simulink library "LIB_TF_G_112"  (Simulink 8.6)
settings: Solver=ode45  StartTime=0.0  StopTime=10.0  RelTol=1e-3
PreLoadFcn:
  | if exist('tl_preloadfcn','file'), tl_preloadfcn(gcs,402); end
PostLoadFcn:
  | if exist('tl_postloadfcn','file'), tl_postloadfcn(gcs,402); end
undefined symbols (not defined in the file): ddv, u2, u3
libraries: tllib x3
(part 3 of 4)

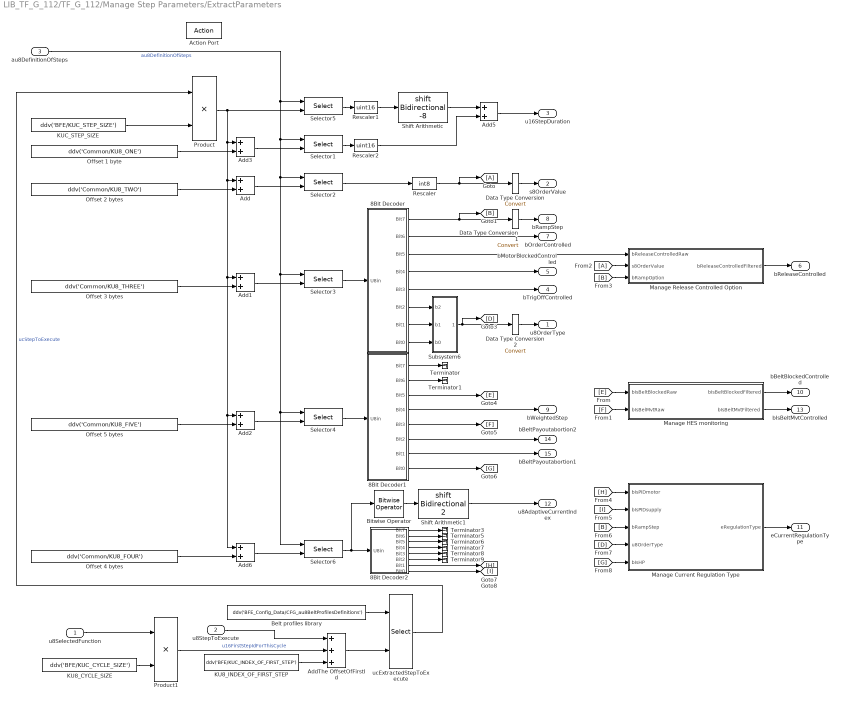
== system LIB_TF_G_112/TF_G_112/Manage Step Parameters/ExtractParameters ==
  u8SelectedFunction : Inport
  u8StepToExecute : Inport  Port=2
  au8DefinitionOfSteps : Inport  RequirementInfo={} %GIDa_5af58792_1cc9_4ce4_bae0_9036b424a801  Port=3
  Action Port : ActionPort  RequirementInfo={} %GIDa_b716945c_1562_44da_9f85_7ecf343fa6e8
  8Bit Decoder : Subsystem  RequirementInfo={} %GIDa_feba0c62_931c_4072_b0ff_45aba4007524  mask(TLSAMPLES_8BIT_DECODER){}
      mask help:
      | Decodes one UInt8 byte into 8 bits.
      | All inputs are boolean variables.
      |
      | Sample implementation using TargetLink Custom Code block.
      | Version 1.0.
  8Bit Decoder1 : Subsystem  RequirementInfo={} %GIDa_d8b7cbf2_0e68_4179_ae19_c2248359c39e  mask(TLSAMPLES_8BIT_DECODER){}
      mask help:
      | Decodes one UInt8 byte into 8 bits.
      | All inputs are boolean variables.
      |
      | Sample implementation using TargetLink Custom Code block.
      | Version 1.0.
  8Bit Decoder2 : Subsystem  RequirementInfo={} %GIDa_1ebe05c3_ad94_48a6_9eed_8520aa55f6d4  mask(TLSAMPLES_8BIT_DECODER){}
      mask help:
      | Decodes one UInt8 byte into 8 bits.
      | All inputs are boolean variables.
      |
      | Sample implementation using TargetLink Custom Code block.
      | Version 1.0.
  Add : Sum  RequirementInfo={} %GIDa_0a57a462_dd82_4f66_b861_c0720a7e3696  mask(TL_Sum){data={'output',{'name','u16StepByte2','type','UInt16'},'date',735951.66828546301}}
      settings: CopyFcn=if exist('tl_reset_reviewflag','file')==2,tl_reset_reviewflag(gcbh);end  DeleteFcn=if exist('delete_tlblock','file')==2,delete_tlblock(gcbh);end  NameChangeFcn=if exist('rename_tlblock','file')==2,rename_tlblock(gcbh);end  OpenFcn=if exist('tl_open_blockdlg','file')==2,tl_open_blockdlg(gcbh);else,open_system(gcbh,'parameter');end
      mask Help: eval(['if exist(''tl_online_help'',''file'') == 2, tl_online_help(''Topic'',''TL_Sum''),else, web([''jar:file:///'',matlabroot,''/help/toolbox/simulink/help.jar!/slref/' lower(get_param(gcbh,'Blocktype')) '.html''], ''-helpbrowser''),end'])
      mask Display: plot([-0.05, 1.05, NaN, -0.05, 1.05],[.01, .01, NaN, .99, .99])
  Add1 : Sum  RequirementInfo={} %GIDa_51ab638f_d75f_42d5_a1b3_c6f4ae26db52  mask(TL_Sum){data={'output',{'name','u16StepByte3','type','UInt16'},'date',735951.66828510421}}
      settings: CopyFcn=if exist('tl_reset_reviewflag','file')==2,tl_reset_reviewflag(gcbh);end  DeleteFcn=if exist('delete_tlblock','file')==2,delete_tlblock(gcbh);end  NameChangeFcn=if exist('rename_tlblock','file')==2,rename_tlblock(gcbh);end  OpenFcn=if exist('tl_open_blockdlg','file')==2,tl_open_blockdlg(gcbh);else,open_system(gcbh,'parameter');end
      mask Help: eval(['if exist(''tl_online_help'',''file'') == 2, tl_online_help(''Topic'',''TL_Sum''),else, web([''jar:file:///'',matlabroot,''/help/toolbox/simulink/help.jar!/slref/' lower(get_param(gcbh,'Blocktype')) '.html''], ''-helpbrowser''),end'])
      mask Display: plot([-0.05, 1.05, NaN, -0.05, 1.05],[.01, .01, NaN, .99, .99])
  Add2 : Sum  RequirementInfo={} %GIDa_81f2c18e_91ec_4878_8faa_bc376be4849a  mask(TL_Sum){data={'output',{'name','u16StepByte5','type','UInt16'},'date',735951.66828473378}}
      settings: CopyFcn=if exist('tl_reset_reviewflag','file')==2,tl_reset_reviewflag(gcbh);end  DeleteFcn=if exist('delete_tlblock','file')==2,delete_tlblock(gcbh);end  NameChangeFcn=if exist('rename_tlblock','file')==2,rename_tlblock(gcbh);end  OpenFcn=if exist('tl_open_blockdlg','file')==2,tl_open_blockdlg(gcbh);else,open_system(gcbh,'parameter');end
      mask Help: eval(['if exist(''tl_online_help'',''file'') == 2, tl_online_help(''Topic'',''TL_Sum''),else, web([''jar:file:///'',matlabroot,''/help/toolbox/simulink/help.jar!/slref/' lower(get_param(gcbh,'Blocktype')) '.html''], ''-helpbrowser''),end'])
      mask Display: plot([-0.05, 1.05, NaN, -0.05, 1.05],[.01, .01, NaN, .99, .99])
  Add3 : Sum  RequirementInfo={} %GIDa_b8557759_ab8c_4963_8e82_441dee7d1691  mask(TL_Sum){data={'output',{'name','u16StepByte1','type','UInt16'},'date',735951.66828436346}}
      settings: CopyFcn=if exist('tl_reset_reviewflag','file')==2,tl_reset_reviewflag(gcbh);end  DeleteFcn=if exist('delete_tlblock','file')==2,delete_tlblock(gcbh);end  NameChangeFcn=if exist('rename_tlblock','file')==2,rename_tlblock(gcbh);end  OpenFcn=if exist('tl_open_blockdlg','file')==2,tl_open_blockdlg(gcbh);else,open_system(gcbh,'parameter');end
      mask Help: eval(['if exist(''tl_online_help'',''file'') == 2, tl_online_help(''Topic'',''TL_Sum''),else, web([''jar:file:///'',matlabroot,''/help/toolbox/simulink/help.jar!/slref/' lower(get_param(gcbh,'Blocktype')) '.html''], ''-helpbrowser''),end'])
      mask Display: plot([-0.05, 1.05, NaN, -0.05, 1.05],[.01, .01, NaN, .99, .99])
  Add5 : Sum  Description=Requirement Titi  RequirementInfo={'other' '..\..\..\..\Documents and Settings\cedric.sauvage\Desktop\BFE_Design.doc' '@Simulink_requirement_item_2' 'true' 'DSG_BFE_00026' '' } %GIDa_05628d3b_8b03_4e96_b55e_ea34f4ea1d4e  AccumDataTypeStr=uint16  OutDataTypeStr=uint16  mask(TL_Sum){data={'comment',{'text',['[COVERS: DSG_BFE_00026]'],'placement',2},'output',{'type','UInt16'},'date',735951.6682839815}}
      settings: CopyFcn=if exist('tl_reset_reviewflag','file')==2,tl_reset_reviewflag(gcbh);end  DeleteFcn=if exist('delete_tlblock','file')==2,delete_tlblock(gcbh);end  NameChangeFcn=if exist('rename_tlblock','file')==2,rename_tlblock(gcbh);end  OpenFcn=if exist('tl_open_blockdlg','file')==2,tl_open_blockdlg(gcbh);else,open_system(gcbh,'parameter');end
      mask Help: eval(['if exist(''tl_online_help'',''file'') == 2, tl_online_help(''Topic'',''TL_Sum''),else, web([''jar:file:///'',matlabroot,''/help/toolbox/simulink/help.jar!/slref/' lower(get_param(gcbh,'Blocktype')) '.html''], ''-helpbrowser''),end'])
      mask Display: plot([-0.05, 1.05, NaN, -0.05, 1.05],[.01, .01, NaN, .99, .99])
  Add6 : Sum  RequirementInfo={} %GIDa_a90a7fc2_4cf2_40a8_9795_cd5c47b64498  mask(TL_Sum){data={'output',{'name','u16StepByte4','type','UInt16'},'date',735951.66828361107}}
      settings: CopyFcn=if exist('tl_reset_reviewflag','file')==2,tl_reset_reviewflag(gcbh);end  DeleteFcn=if exist('delete_tlblock','file')==2,delete_tlblock(gcbh);end  NameChangeFcn=if exist('rename_tlblock','file')==2,rename_tlblock(gcbh);end  OpenFcn=if exist('tl_open_blockdlg','file')==2,tl_open_blockdlg(gcbh);else,open_system(gcbh,'parameter');end
      mask Help: eval(['if exist(''tl_online_help'',''file'') == 2, tl_online_help(''Topic'',''TL_Sum''),else, web([''jar:file:///'',matlabroot,''/help/toolbox/simulink/help.jar!/slref/' lower(get_param(gcbh,'Blocktype')) '.html''], ''-helpbrowser''),end'])
      mask Display: plot([-0.05, 1.05, NaN, -0.05, 1.05],[.01, .01, NaN, .99, .99])
  AddThe OffsetOfFirstId : Sum  RequirementInfo={} %GIDa_cb935c7f_f3b5_47b3_8f86_966f4978fe65  Inputs=+++  SaturateOnIntegerOverflow=on  OutDataTypeStr=Inherit: Same as first input  mask(TL_Sum){data={'output',{'name','u16StepBytePosition','class','MERGEABLE_GLOBAL_ASR4','type','UInt16'},'date',736468.40163105319}}
      settings: CopyFcn=if exist('tl_reset_reviewflag','file')==2,tl_reset_reviewflag(gcbh);end  DeleteFcn=if exist('delete_tlblock','file')==2,delete_tlblock(gcbh);end  NameChangeFcn=if exist('rename_tlblock','file')==2,rename_tlblock(gcbh);end  OpenFcn=if exist('tl_open_blockdlg','file')==2,tl_open_blockdlg(gcbh);else,open_system(gcbh,'parameter');end
      mask Help: eval(['if exist(''tl_online_help'',''file'') == 2, tl_online_help(''Topic'',''TL_Sum''),else, web([''jar:file:///'',matlabroot,''/help/toolbox/simulink/help.jar!/slref/' lower(get_param(gcbh,'Blocktype')) '.html''], ''-helpbrowser''),end'])
      mask Display: plot([-0.05, 1.05, NaN, -0.05, 1.05],[.01, .01, NaN, .99, .99])
  Belt profiles library : Constant  RequirementInfo={} %GIDa_12d42078_1b0f_4eb4_abcd_54e33e78707a  Value=ddv('BFE_Config_Data/CFG_au8BeltProfilesDefinitions')  OutDataTypeStr=uint8  SampleTime=-1  mask(TL_Constant){data={'output',{'variable','BFE_Config_Data/CFG_au8BeltProfilesDefinitions'},'autoscaling',{'mode',2,'scalingvalid',1},'date',735951.66828289349}}
      settings: CopyFcn=if exist('tl_reset_reviewflag','file')==2,tl_reset_reviewflag(gcbh);end  DeleteFcn=if exist('delete_tlblock','file')==2,delete_tlblock(gcbh);end  NameChangeFcn=if exist('rename_tlblock','file')==2,rename_tlblock(gcbh);end  OpenFcn=if exist('tl_open_blockdlg','file')==2,tl_open_blockdlg(gcbh);else,open_system(gcbh,'parameter');end
      mask Help: eval(['if exist(''tl_online_help'',''file'') == 2, tl_online_help(''Topic'',''TL_Constant''),else, web([''jar:file:///'',matlabroot,''/help/toolbox/simulink/help.jar!/slref/' lower(get_param(gcbh,'Blocktype')) '.html''], ''-helpbrowser''),end'])
      mask Display: plot([-0.05, 1.05, NaN, -0.05, 1.05],[.01, .01, NaN, .99, .99])
  Bitwise Operator : tllib/Bitwise Operator  logicop=AND  UseBitMask=on  BitMask=bin2dec('11111100')  BitMaskRealWorld=Stored Integer  data={'bitmask',{'variable','Common/KU8_MASK_BITS_2_7'},'date',735951.66828241898}
  Data Type Conversion : DataTypeConversion
  Data Type Conversion1 : DataTypeConversion
  Data Type Conversion2 : DataTypeConversion
  KU8_CYCLE_SIZE : Constant  RequirementInfo={} %GIDa_f33bf5cd_925c_4e93_b1c0_651200f97367  Value=ddv('BFE/KUC_CYCLE_SIZE')  OutDataTypeStr=Inherit: Inherit via back propagation  mask(TL_Constant){data={'output',{'variable','BFE/KUC_CYCLE_SIZE'},'date',735951.66828206019}}
      settings: CopyFcn=if exist('tl_reset_reviewflag','file')==2,tl_reset_reviewflag(gcbh);end  DeleteFcn=if exist('delete_tlblock','file')==2,delete_tlblock(gcbh);end  NameChangeFcn=if exist('rename_tlblock','file')==2,rename_tlblock(gcbh);end  OpenFcn=if exist('tl_open_blockdlg','file')==2,tl_open_blockdlg(gcbh);else,open_system(gcbh,'parameter');end
      mask Help: eval(['if exist(''tl_online_help'',''file'') == 2, tl_online_help(''Topic'',''TL_Constant''),else, web([''jar:file:///'',matlabroot,''/help/toolbox/simulink/help.jar!/slref/' lower(get_param(gcbh,'Blocktype')) '.html''], ''-helpbrowser''),end'])
      mask Display: plot([-0.05, 1.05, NaN, -0.05, 1.05],[.01, .01, NaN, .99, .99])
  KU8_INDEX_OF_FIRST_STEP : Constant  RequirementInfo={} %GIDa_c9f92c82_efc8_46a4_b98e_26be3633ccb9  Value=ddv('BFE/KUC_INDEX_OF_FIRST_STEP')  OutDataTypeStr=Inherit: Inherit via back propagation  mask(TL_Constant){data={'output',{'variable','BFE/KUC_INDEX_OF_FIRST_STEP'},'date',735951.66828170139}}
      settings: CopyFcn=if exist('tl_reset_reviewflag','file')==2,tl_reset_reviewflag(gcbh);end  DeleteFcn=if exist('delete_tlblock','file')==2,delete_tlblock(gcbh);end  NameChangeFcn=if exist('rename_tlblock','file')==2,rename_tlblock(gcbh);end  OpenFcn=if exist('tl_open_blockdlg','file')==2,tl_open_blockdlg(gcbh);else,open_system(gcbh,'parameter');end
      mask Help: eval(['if exist(''tl_online_help'',''file'') == 2, tl_online_help(''Topic'',''TL_Constant''),else, web([''jar:file:///'',matlabroot,''/help/toolbox/simulink/help.jar!/slref/' lower(get_param(gcbh,'Blocktype')) '.html''], ''-helpbrowser''),end'])
      mask Display: plot([-0.05, 1.05, NaN, -0.05, 1.05],[.01, .01, NaN, .99, .99])
  KUC_STEP_SIZE : Constant  RequirementInfo={} %GIDa_b75dc5a3_ad3f_404e_b74d_edddff931102  Value=ddv('BFE/KUC_STEP_SIZE')  OutDataTypeStr=Inherit: Inherit via back propagation  SampleTime=-1  mask(TL_Constant){data={'output',{'variable','BFE/KUC_STEP_SIZE'},'date',735951.6682813426}}
      settings: CopyFcn=if exist('tl_reset_reviewflag','file')==2,tl_reset_reviewflag(gcbh);end  DeleteFcn=if exist('delete_tlblock','file')==2,delete_tlblock(gcbh);end  NameChangeFcn=if exist('rename_tlblock','file')==2,rename_tlblock(gcbh);end  OpenFcn=if exist('tl_open_blockdlg','file')==2,tl_open_blockdlg(gcbh);else,open_system(gcbh,'parameter');end
      mask Help: eval(['if exist(''tl_online_help'',''file'') == 2, tl_online_help(''Topic'',''TL_Constant''),else, web([''jar:file:///'',matlabroot,''/help/toolbox/simulink/help.jar!/slref/' lower(get_param(gcbh,'Blocktype')) '.html''], ''-helpbrowser''),end'])
      mask Display: plot([-0.05, 1.05, NaN, -0.05, 1.05],[.01, .01, NaN, .99, .99])
  Manage Current Regulation Type : Subsystem  TreatAsAtomicUnit=on
  Manage HES monitoring : Subsystem  TreatAsAtomicUnit=on
  Manage Release Controlled Option : Subsystem  TreatAsAtomicUnit=on
  Offset 1 byte : Constant  RequirementInfo={} %GIDa_3a3d9ef6_6e74_4523_8795_3102c60b89ad  Value=ddv('Common/KU8_ONE')  OutDataTypeStr=uint8  SampleTime=-1  mask(TL_Constant){data={'output',{'variable','Common/KU8_ONE'},'date',735951.66827084485}}
      settings: CopyFcn=if exist('tl_reset_reviewflag','file')==2,tl_reset_reviewflag(gcbh);end  DeleteFcn=if exist('delete_tlblock','file')==2,delete_tlblock(gcbh);end  NameChangeFcn=if exist('rename_tlblock','file')==2,rename_tlblock(gcbh);end  OpenFcn=if exist('tl_open_blockdlg','file')==2,tl_open_blockdlg(gcbh);else,open_system(gcbh,'parameter');end
      mask Help: eval(['if exist(''tl_online_help'',''file'') == 2, tl_online_help(''Topic'',''TL_Constant''),else, web([''jar:file:///'',matlabroot,''/help/toolbox/simulink/help.jar!/slref/' lower(get_param(gcbh,'Blocktype')) '.html''], ''-helpbrowser''),end'])
      mask Display: plot([-0.05, 1.05, NaN, -0.05, 1.05],[.01, .01, NaN, .99, .99])
  Offset 2 bytes : Constant  RequirementInfo={} %GIDa_19184c90_6870_45c3_8db8_a8942b4be325  Value=ddv('Common/KU8_TWO')  OutDataTypeStr=uint8  SampleTime=-1  mask(TL_Constant){data={'output',{'variable','Common/KU8_TWO'},'date',735951.66827048606}}
      settings: CopyFcn=if exist('tl_reset_reviewflag','file')==2,tl_reset_reviewflag(gcbh);end  DeleteFcn=if exist('delete_tlblock','file')==2,delete_tlblock(gcbh);end  NameChangeFcn=if exist('rename_tlblock','file')==2,rename_tlblock(gcbh);end  OpenFcn=if exist('tl_open_blockdlg','file')==2,tl_open_blockdlg(gcbh);else,open_system(gcbh,'parameter');end
      mask Help: eval(['if exist(''tl_online_help'',''file'') == 2, tl_online_help(''Topic'',''TL_Constant''),else, web([''jar:file:///'',matlabroot,''/help/toolbox/simulink/help.jar!/slref/' lower(get_param(gcbh,'Blocktype')) '.html''], ''-helpbrowser''),end'])
      mask Display: plot([-0.05, 1.05, NaN, -0.05, 1.05],[.01, .01, NaN, .99, .99])
  Offset 3 bytes : Constant  RequirementInfo={} %GIDa_4ca9dd1f_f166_4945_8d3c_5d2b0f97e3a1  Value=ddv('Common/KU8_THREE')  OutDataTypeStr=uint8  SampleTime=-1  mask(TL_Constant){data={'output',{'variable','Common/KU8_THREE'},'date',735951.66827010422}}
      settings: CopyFcn=if exist('tl_reset_reviewflag','file')==2,tl_reset_reviewflag(gcbh);end  DeleteFcn=if exist('delete_tlblock','file')==2,delete_tlblock(gcbh);end  NameChangeFcn=if exist('rename_tlblock','file')==2,rename_tlblock(gcbh);end  OpenFcn=if exist('tl_open_blockdlg','file')==2,tl_open_blockdlg(gcbh);else,open_system(gcbh,'parameter');end
      mask Help: eval(['if exist(''tl_online_help'',''file'') == 2, tl_online_help(''Topic'',''TL_Constant''),else, web([''jar:file:///'',matlabroot,''/help/toolbox/simulink/help.jar!/slref/' lower(get_param(gcbh,'Blocktype')) '.html''], ''-helpbrowser''),end'])
      mask Display: plot([-0.05, 1.05, NaN, -0.05, 1.05],[.01, .01, NaN, .99, .99])
  Offset 4 bytes : Constant  RequirementInfo={} %GIDa_ea66cbc1_e91d_4821_b668_d6b79850c644  Value=ddv('Common/KU8_FOUR')  OutDataTypeStr=uint8  SampleTime=-1  mask(TL_Constant){data={'output',{'variable','Common/KU8_FOUR'},'date',735951.66826973378}}
      settings: CopyFcn=if exist('tl_reset_reviewflag','file')==2,tl_reset_reviewflag(gcbh);end  DeleteFcn=if exist('delete_tlblock','file')==2,delete_tlblock(gcbh);end  NameChangeFcn=if exist('rename_tlblock','file')==2,rename_tlblock(gcbh);end  OpenFcn=if exist('tl_open_blockdlg','file')==2,tl_open_blockdlg(gcbh);else,open_system(gcbh,'parameter');end
      mask Help: eval(['if exist(''tl_online_help'',''file'') == 2, tl_online_help(''Topic'',''TL_Constant''),else, web([''jar:file:///'',matlabroot,''/help/toolbox/simulink/help.jar!/slref/' lower(get_param(gcbh,'Blocktype')) '.html''], ''-helpbrowser''),end'])
      mask Display: plot([-0.05, 1.05, NaN, -0.05, 1.05],[.01, .01, NaN, .99, .99])
  Offset 5 bytes : Constant  RequirementInfo={} %GIDa_d7e3fc43_2c8c_428d_9f27_caf2b47de596  Value=ddv('Common/KU8_FIVE')  OutDataTypeStr=uint8  SampleTime=-1  mask(TL_Constant){data={'output',{'variable','Common/KU8_FIVE'},'date',735951.66826935182}}
      settings: CopyFcn=if exist('tl_reset_reviewflag','file')==2,tl_reset_reviewflag(gcbh);end  DeleteFcn=if exist('delete_tlblock','file')==2,delete_tlblock(gcbh);end  NameChangeFcn=if exist('rename_tlblock','file')==2,rename_tlblock(gcbh);end  OpenFcn=if exist('tl_open_blockdlg','file')==2,tl_open_blockdlg(gcbh);else,open_system(gcbh,'parameter');end
      mask Help: eval(['if exist(''tl_online_help'',''file'') == 2, tl_online_help(''Topic'',''TL_Constant''),else, web([''jar:file:///'',matlabroot,''/help/toolbox/simulink/help.jar!/slref/' lower(get_param(gcbh,'Blocktype')) '.html''], ''-helpbrowser''),end'])
      mask Display: plot([-0.05, 1.05, NaN, -0.05, 1.05],[.01, .01, NaN, .99, .99])
  Product : Product  RequirementInfo={} %GIDa_7eb561e5_5106_47b1_bccb_d25d321f907e  OutDataTypeStr=uint16  RndMeth=Zero  mask(TL_Product){data={'output',{'name','u16StepByte0','class','MERGEABLE_GLOBAL_ASR4','type','UInt16'},'date',736468.39839604171}}
      settings: CopyFcn=if exist('tl_reset_reviewflag','file')==2,tl_reset_reviewflag(gcbh);end  DeleteFcn=if exist('delete_tlblock','file')==2,delete_tlblock(gcbh);end  NameChangeFcn=if exist('rename_tlblock','file')==2,rename_tlblock(gcbh);end  OpenFcn=if exist('tl_open_blockdlg','file')==2,tl_open_blockdlg(gcbh);else,open_system(gcbh,'parameter');end
      mask Help: eval(['if exist(''tl_online_help'',''file'') == 2, tl_online_help(''Topic'',''TL_Product''),else, web([''jar:file:///'',matlabroot,''/help/toolbox/simulink/help.jar!/slref/' lower(get_param(gcbh,'Blocktype')) '.html''], ''-helpbrowser''),end'])
      mask Display: plot([-0.05, 1.05, NaN, -0.05, 1.05],[.01, .01, NaN, .99, .99])
  Product1 : Product  RequirementInfo={} %GIDa_7bc72bc7_7488_430d_ac37_90a0b87b4fce  SaturateOnIntegerOverflow=on  RndMeth=Zero  mask(TL_Product){data={'output',{'type','UInt16'},'date',735951.66826856486}}
      settings: CopyFcn=if exist('tl_reset_reviewflag','file')==2,tl_reset_reviewflag(gcbh);end  DeleteFcn=if exist('delete_tlblock','file')==2,delete_tlblock(gcbh);end  NameChangeFcn=if exist('rename_tlblock','file')==2,rename_tlblock(gcbh);end  OpenFcn=if exist('tl_open_blockdlg','file')==2,tl_open_blockdlg(gcbh);else,open_system(gcbh,'parameter');end
      mask Help: eval(['if exist(''tl_online_help'',''file'') == 2, tl_online_help(''Topic'',''TL_Product''),else, web([''jar:file:///'',matlabroot,''/help/toolbox/simulink/help.jar!/slref/' lower(get_param(gcbh,'Blocktype')) '.html''], ''-helpbrowser''),end'])
      mask Display: plot([-0.05, 1.05, NaN, -0.05, 1.05],[.01, .01, NaN, .99, .99])
  Rescaler : DataTypeConversion  RequirementInfo={'other' '..\..\..\..\Documents and Settings\cedric.sauvage\Desktop\BFE_Design.doc' '@Simulink_requirement_item_3' 'true' 'DSG_BFE_00025' '' } %GIDa_58362dca_0e5a_418f_af47_1f6b1fc37d26  OutDataTypeStr=int8  RndMeth=Zero  mask(TL_Rescaler){data={'comment',{'text',['[COVERS: DSG_BFE_00025]'],'placement',2},'output',{'name','s8StepOrderValue','type','Int8'},'date',735951.66826821759}}
      settings: DeleteFcn=if exist('delete_tlblock','file')==2,delete_tlblock(gcbh);end  NameChangeFcn=if exist('rename_tlblock','file')==2,rename_tlblock(gcbh);end  OpenFcn=if exist('tl_open_blockdlg','file')==2,tl_open_blockdlg(gcbh);else,open_system(gcbh,'parameter');end
      mask Help: eval(['if exist(''tl_online_help'',''file'') == 2, tl_online_help(''Topic'',''TL_Rescaler''),else, web([''jar:file:///'',matlabroot,''/help/toolbox/simulink/help.jar!/slref/' lower(get_param(gcbh,'Blocktype')) '.html''], ''-helpbrowser''),end'])
      mask Display: plot([-0.05, 1.05, NaN, -0.05, 1.05],[.01, .01, NaN, .99, .99])
  Rescaler1 : DataTypeConversion  OutDataTypeStr=uint16  SaturateOnIntegerOverflow=on  RndMeth=Zero  mask(TL_Rescaler){data={'output',{'type','UInt16'},'date',735951.66826790513}}
      settings: DeleteFcn=if exist('delete_tlblock','file')==2,delete_tlblock(gcbh);end  NameChangeFcn=if exist('rename_tlblock','file')==2,rename_tlblock(gcbh);end  OpenFcn=if exist('tl_open_blockdlg','file')==2,tl_open_blockdlg(gcbh);else,open_system(gcbh,'parameter');end
      mask Help: eval(['if exist(''tl_online_help'',''file'') == 2, tl_online_help(''Topic'',''TL_Rescaler''),else, web([''jar:file:///'',matlabroot,''/help/toolbox/simulink/help.jar!/slref/' lower(get_param(gcbh,'Blocktype')) '.html''], ''-helpbrowser''),end'])
      mask Display: plot([-0.05, 1.05, NaN, -0.05, 1.05],[.01, .01, NaN, .99, .99])
  Rescaler2 : DataTypeConversion  OutDataTypeStr=uint16  SaturateOnIntegerOverflow=on  RndMeth=Zero  mask(TL_Rescaler){data={'output',{'type','UInt16'},'date',735951.66826758103}}
      settings: DeleteFcn=if exist('delete_tlblock','file')==2,delete_tlblock(gcbh);end  NameChangeFcn=if exist('rename_tlblock','file')==2,rename_tlblock(gcbh);end  OpenFcn=if exist('tl_open_blockdlg','file')==2,tl_open_blockdlg(gcbh);else,open_system(gcbh,'parameter');end
      mask Help: eval(['if exist(''tl_online_help'',''file'') == 2, tl_online_help(''Topic'',''TL_Rescaler''),else, web([''jar:file:///'',matlabroot,''/help/toolbox/simulink/help.jar!/slref/' lower(get_param(gcbh,'Blocktype')) '.html''], ''-helpbrowser''),end'])
      mask Display: plot([-0.05, 1.05, NaN, -0.05, 1.05],[.01, .01, NaN, .99, .99])
  Selector1 : Selector  RequirementInfo={} %GIDa_4422b87b_5746_46e1_a326_9d16cdd82f03  IndexMode=Zero-based  IndexOptions=Index vector (port)  Indices=[1:10]  OutputSizes=1
  Selector2 : Selector  RequirementInfo={} %GIDa_4d9cfe24_d7c1_4186_b1de_afe3f89ce847  IndexMode=Zero-based  IndexOptions=Index vector (port)  Indices=[1:10]  OutputSizes=1
  Selector3 : Selector  RequirementInfo={} %GIDa_709804a5_dd5b_4c61_8f3f_1a0b2ad04ecf  IndexMode=Zero-based  IndexOptions=Index vector (port)  Indices=[1:10]  OutputSizes=1
  Selector4 : Selector  RequirementInfo={} %GIDa_f598d6e8_f893_4a7f_8905_585de03faa36  IndexMode=Zero-based  IndexOptions=Index vector (port)  Indices=[1:10]  OutputSizes=1
  Selector5 : Selector  RequirementInfo={} %GIDa_dd185a0d_3844_4a34_af71_6fb5e1e75326  IndexMode=Zero-based  IndexOptions=Index vector (port)  Indices=[1:10]  OutputSizes=1
  Selector6 : Selector  RequirementInfo={} %GIDa_61c5be39_750f_4521_8022_d14d6bd83ead  IndexMode=Zero-based  IndexOptions=Index vector (port)  Indices=[1:10]  OutputSizes=1
  Shift Arithmetic : ArithShift  LoadFcn=hBlOcK = gcbh; if strcmp(get_param(hBlOcK, 'LinkStatus'), 'resolved'), set_param(hBlOcK, 'LinkStatus', 'none'); set_param(hBlOcK, 'LoadFcn', ''); end; clear('hBlOcK');  BitShiftNumber=-8  mask(TL_ArithShift){data={'date',735951.66826726857}}
      settings: DeleteFcn=if exist('delete_tlblock','file')==2,delete_tlblock(gcbh);end  NameChangeFcn=if exist('rename_tlblock','file')==2,rename_tlblock(gcbh);end  OpenFcn=if exist('tl_open_blockdlg','file')==2,tl_open_blockdlg(gcbh);else,open_system(gcbh,'parameter');end
      mask Help: eval(['if exist(''tl_online_help'',''file'') == 2, tl_online_help(''Topic'',''TL_ArithShift''),else, web([''jar:file:///'',matlabroot,''/help/toolbox/simulink/help.jar!/slref/' lower(get_param(gcbh,'Blocktype')) '.html''], ''-helpbrowser''),end'])
      mask Display: plot([-0.05, 1.05, NaN, -0.05, 1.05],[.01, .01, NaN, .99, .99])
  Shift Arithmetic1 : ArithShift  LoadFcn=hBlOcK = gcbh; if strcmp(get_param(hBlOcK, 'LinkStatus'), 'resolved'), set_param(hBlOcK, 'LinkStatus', 'none'); set_param(hBlOcK, 'LoadFcn', ''); end; clear('hBlOcK');  BitShiftNumber=2  mask(TL_ArithShift){data={'date',735951.66826699069}}
      settings: DeleteFcn=if exist('delete_tlblock','file')==2,delete_tlblock(gcbh);end  NameChangeFcn=if exist('rename_tlblock','file')==2,rename_tlblock(gcbh);end  OpenFcn=if exist('tl_open_blockdlg','file')==2,tl_open_blockdlg(gcbh);else,open_system(gcbh,'parameter');end
      mask Help: eval(['if exist(''tl_online_help'',''file'') == 2, tl_online_help(''Topic'',''TL_ArithShift''),else, web([''jar:file:///'',matlabroot,''/help/toolbox/simulink/help.jar!/slref/' lower(get_param(gcbh,'Blocktype')) '.html''], ''-helpbrowser''),end'])
      mask Display: plot([-0.05, 1.05, NaN, -0.05, 1.05],[.01, .01, NaN, .99, .99])
  Subsystem6 : Subsystem  RequirementInfo={} %GIDa_5160330e_cdd9_425d_8875_f8236145217b
  Terminator{,1,3,5..9} (8 alike) : Terminator
      Terminator settings: RequirementInfo={} %GIDa_d177cf0d_d072_4e9c_ab8a_78740cfb15e6
      Terminator1 settings: RequirementInfo={} %GIDa_be300696_ad1a_42f1_b0f4_805d67844eb4
      Terminator3 settings: RequirementInfo={} %GIDa_1a9de90a_a8b4_48de_855e_2f833ecb0368
      Terminator5 settings: RequirementInfo={} %GIDa_bf4837d6_3514_42e9_b333_5cacb99f9262
      Terminator6 settings: RequirementInfo={} %GIDa_fb26de38_7835_46a8_84f0_dac9813e6326
      Terminator7 settings: RequirementInfo={} %GIDa_a50c1da3_624f_4d2f_b153_1f4068f0cf80
      Terminator8 settings: RequirementInfo={} %GIDa_7348f082_2a2a_40ba_aa6f_788e86812770
      Terminator9 settings: RequirementInfo={} %GIDa_ebf10ede_7946_4cab_8c57_47c6be569568
  ucExtractedStepToExecute : Selector  RequirementInfo={} %GIDa_d02645cd_0f6b_42d4_ae8b_fb6bc63cfc7b  IndexMode=Zero-based  IndexOptions=Index vector (port)  Indices=[1:3]  OutputSizes=1
  u8OrderType : Outport  RequirementInfo={} %GIDa_a4ff17c9_84cc_43ee_8b0c_3fd6b6f1ed09  InitialOutput=7
  s8OrderValue : Outport  RequirementInfo={} %GIDa_36792c2a_0fa2_493d_8829_1fb3067ac82d  Port=2  InitialOutput=0
  u16StepDuration : Outport  RequirementInfo={} %GIDa_e6c8acc4_bf57_4474_843a_d9aa89ac3819  Port=3  InitialOutput=0
  bTrigOffControlled : Outport  RequirementInfo={} %GIDa_3fe998c0_2753_48e9_84d2_02b12f72de18  Port=4  InitialOutput=0
  bMotorBlockedControlled : Outport  RequirementInfo={} %GIDa_a830c711_4505_4102_b674_229ec271b529  Port=5  InitialOutput=0
  bReleaseControlled : Outport  RequirementInfo={} %GIDa_8c367dcb_6d8d_4602_bfad_447b7cbcf509  Port=6  InitialOutput=0
  bOrderControlled : Outport  RequirementInfo={} %GIDa_2d51edae_6320_46d1_8886_e073955a6cde  Port=7  InitialOutput=0
  bRampStep : Outport  RequirementInfo={} %GIDa_14c0e694_bffc_4663_9ef2_68c7701718bc  Port=8  InitialOutput=0
  bWeightedStep : Outport  RequirementInfo={} %GIDa_281ae594_fd74_4bf7_8434_defd59967c3f  Port=9  InitialOutput=0
  bBeltBlockedControlled : Outport  RequirementInfo={} %GIDa_83e772d5_3502_473a_b2ff_7f8717149afd  Port=10  InitialOutput=0
  eCurrentRegulationType : Outport  RequirementInfo={} %GIDa_6e2b43b7_4cdb_437c_82fa_b7a637421221  Port=11  InitialOutput=0
  u8AdaptiveCurrentIndex : Outport  RequirementInfo={} %GIDa_738e03a2_16a7_4117_b6a7_daaa152fa532  Port=12  InitialOutput=0
  bIsBeltMvtControlled : Outport  RequirementInfo={} %GIDa_b6401444_b6f7_48ef_967a_cafed8a8d51a  Port=13  InitialOutput=0
  bBeltPayoutabortion2 : Outport  RequirementInfo={} %GIDa_dece0d12_f4b9_48c5_8979_e98e0f3f5575  Port=14  InitialOutput=0
  bBeltPayoutabortion1 : Outport  RequirementInfo={} %GIDa_1df73305_fc6f_4d9e_8545_b92e5439accf  Port=15  InitialOutput=0
  wires:
  Shift Arithmetic1/1 -> u8AdaptiveCurrentIndex/1
  8Bit Decoder2/8(Bit0) -> [I]
  8Bit Decoder2/7(Bit1) -> [H]
  Selector6/1 -> 8Bit Decoder2/1(U8in), Bitwise Operator/1
  Offset 4 bytes/1 -> Add6/2
  Add6/1 -> Selector6/2
  8Bit Decoder1/8(Bit0) -> [G]
  8Bit Decoder1/7(Bit1) -> bBeltPayoutabortion1/1
  8Bit Decoder1/5(Bit3) -> [F]
  8Bit Decoder1/2(Bit6) -> Terminator1/1
  8Bit Decoder1/1(Bit7) -> Terminator/1
  8Bit Decoder1/3(Bit5) -> [E]
  KUC_STEP_SIZE/1 -> Product/2
  ucExtractedStepToExecute/1 -> Product/1  "ucStepToExecute"
  Selector2/1 -> Rescaler/1
  8Bit Decoder/8(Bit0) -> Subsystem6/3(b0)
  8Bit Decoder/7(Bit1) -> Subsystem6/2(b1)
  8Bit Decoder/6(Bit2) -> Subsystem6/1(b2)
  Selector4/1 -> 8Bit Decoder1/1(U8in)
  au8DefinitionOfSteps/1 -> Selector5/1, Selector6/1, Selector4/1, Selector3/1, Selector2/1, Selector1/1  "au8DefinitionOfSteps"
  Add5/1 -> u16StepDuration/1
  Offset 2 bytes/1 -> Add/2
  Selector3/1 -> 8Bit Decoder/1(U8in)
  Subsystem6/1(Out1) -> [D], Data Type Conversion2/1
  8Bit Decoder/5(Bit3) -> bTrigOffControlled/1
  8Bit Decoder/3(Bit5) -> Manage Release Controlled Option/1(bReleaseControlledRaw)
  8Bit Decoder/2(Bit6) -> bOrderControlled/1
  8Bit Decoder/1(Bit7) -> [B], Data Type Conversion1/1
  8Bit Decoder1/4(Bit4) -> bWeightedStep/1
  8Bit Decoder/4(Bit4) -> bMotorBlockedControlled/1
  Rescaler/1 -> [A], Data Type Conversion/1
  Offset 5 bytes/1 -> Add2/2
  Offset 3 bytes/1 -> Add1/2
  Product/1 -> Add/1, Add6/1, Add2/1, Add1/1, Add3/1, Selector5/2
  Add/1 -> Selector2/2
  Add1/1 -> Selector3/2
  Add2/1 -> Selector4/2
  Offset 1 byte/1 -> Add3/2
  Add3/1 -> Selector1/2
  Selector5/1 -> Rescaler1/1
  Shift Arithmetic/1 -> Add5/1
  Selector1/1 -> Rescaler2/1
  8Bit Decoder2/1(Bit7) -> Terminator3/1
  8Bit Decoder2/2(Bit6) -> Terminator5/1
  8Bit Decoder2/3(Bit5) -> Terminator6/1
  8Bit Decoder2/4(Bit4) -> Terminator7/1
  8Bit Decoder2/5(Bit3) -> Terminator8/1
  8Bit Decoder2/6(Bit2) -> Terminator9/1
  8Bit Decoder1/6(Bit2) -> bBeltPayoutabortion2/1
  Rescaler2/1 -> Add5/2
  Rescaler1/1 -> Shift Arithmetic/1
  Bitwise Operator/1 -> Shift Arithmetic1/1
  Manage Release Controlled Option/1(bReleaseControlledFiltered) -> bReleaseControlled/1
  [A] -> Manage Release Controlled Option/2(s8OrderValue)
  [B] -> Manage Release Controlled Option/3(bRampOption)
  Manage HES monitoring/1(bIsBeltBlockedFiltered) -> bBeltBlockedControlled/1
  Manage HES monitoring/2(bIsBeltMvtFiltered) -> bIsBeltMvtControlled/1
  [E] -> Manage HES monitoring/1(bIsBeltBlockedRaw)
  [F] -> Manage HES monitoring/2(bIsBelMvtRaw)
  Data Type Conversion/1 -> s8OrderValue/1
  Data Type Conversion1/1 -> bRampStep/1
  Data Type Conversion2/1 -> u8OrderType/1
  [H] -> Manage Current Regulation Type/1(bIsPIDmotor)
  [I] -> Manage Current Regulation Type/2(bIsPIDsupply)
  [B] -> Manage Current Regulation Type/3(bRampStep)
  [D] -> Manage Current Regulation Type/4(u8OrderType)
  [G] -> Manage Current Regulation Type/5(bIsHP)
  Manage Current Regulation Type/1(eRegulationType) -> eCurrentRegulationType/1
  Product1/1 -> AddThe OffsetOfFirstId/2  "u16FirstStepIdForThisCycle"
  AddThe OffsetOfFirstId/1 -> ucExtractedStepToExecute/2
  KU8_CYCLE_SIZE/1 -> Product1/2
  u8SelectedFunction/1 -> Product1/1
  KU8_INDEX_OF_FIRST_STEP/1 -> AddThe OffsetOfFirstId/3
  u8StepToExecute/1 -> AddThe OffsetOfFirstId/1
  Belt profiles library/1 -> ucExtractedStepToExecute/1

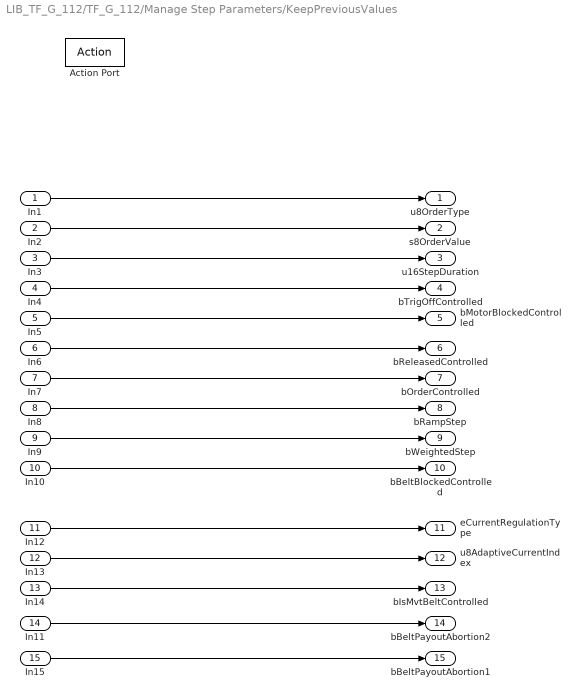
== system LIB_TF_G_112/TF_G_112/Manage Step Parameters/KeepPreviousValues ==
  In1 : Inport  RequirementInfo={} %GIDa_61173a58_4933_4291_992c_59970ace437c
  In2 : Inport  RequirementInfo={} %GIDa_8cf21477_d934_4301_991e_495f48917b5b  Port=2
  In3 : Inport  RequirementInfo={} %GIDa_271bfe5f_683d_4e40_816a_3ac303e31e66  Port=3
  In4 : Inport  RequirementInfo={} %GIDa_6c29d33a_bdf3_4273_9cb2_30a13c55fc11  Port=4
  In5 : Inport  RequirementInfo={} %GIDa_9147d5a5_b635_44da_8129_5490312102e1  Port=5
  In6 : Inport  RequirementInfo={} %GIDa_b8e80f99_6f22_40ff_965f_fd3097931f0c  Port=6
  In7 : Inport  RequirementInfo={} %GIDa_96e19a64_61d9_48fa_bb9c_95181a73e921  Port=7
  In8 : Inport  RequirementInfo={} %GIDa_5931d3fb_f7e2_4f1e_b015_1aa9df9138bb  Port=8
  In9 : Inport  RequirementInfo={} %GIDa_2e1a0281_8b1a_4a62_a6b7_d6f3cbbd3bbf  Port=9
  In10 : Inport  RequirementInfo={} %GIDa_4f39fde8_23e2_4196_929a_01b895998a06  Port=10
  In12 : Inport  RequirementInfo={} %GIDa_506cfe8a_115e_4445_ac9a_915942cdda23  Port=11
  In13 : Inport  RequirementInfo={} %GIDa_c242d6e1_ad36_4cca_b0ff_34cd6fa41a8f  Port=12
  In14 : Inport  RequirementInfo={} %GIDa_56afc156_3db9_454c_89b0_63cf85556edf  Port=13
  In11 : Inport  RequirementInfo={} %GIDa_3281a84f_454f_4950_a479_80382cac1cd2  Port=14
  In15 : Inport  RequirementInfo={} %GIDa_0a0e402d_e062_4179_a70f_2ca17d0be5ed  Port=15
  Action Port : ActionPort  RequirementInfo={} %GIDa_96d1ad58_50a9_4027_a59b_05d48c1814fd
  u8OrderType : Outport  RequirementInfo={} %GIDa_fdafd93d_054e_49a8_b09d_e2e4e30d580e  InitialOutput=7
  s8OrderValue : Outport  RequirementInfo={} %GIDa_357db256_5324_4153_8420_788fb44903fc  Port=2  InitialOutput=0
  u16StepDuration : Outport  RequirementInfo={} %GIDa_92a7c2d2_80da_4891_972c_b6d6040a431b  Port=3  InitialOutput=0
  bTrigOffControlled : Outport  RequirementInfo={} %GIDa_31ffab98_dfe5_4cbe_8309_cfdec138b26b  Port=4  InitialOutput=0
  bMotorBlockedControlled : Outport  RequirementInfo={} %GIDa_f1828f97_0ae8_4691_a044_c353b31799c7  Port=5  InitialOutput=0
  bReleasedControlled : Outport  RequirementInfo={} %GIDa_347eca28_f2d2_4a3b_9baf_2c599b943acb  Port=6  InitialOutput=0
  bOrderControlled : Outport  RequirementInfo={} %GIDa_8edec4cc_6b82_4e60_8bd9_f00fe3e9d9a5  Port=7  InitialOutput=0
  bRampStep : Outport  RequirementInfo={} %GIDa_b542afc9_2a48_4d54_9cbd_42bb43ac3208  Port=8  InitialOutput=0
  bWeightedStep : Outport  RequirementInfo={} %GIDa_ccc30436_643b_422d_ad64_4a42024accfc  Port=9  InitialOutput=0
  bBeltBlockedControlled : Outport  RequirementInfo={} %GIDa_51e91ca6_7004_4a4d_9acd_a737dd3b7a94  Port=10  InitialOutput=0
  eCurrentRegulationType : Outport  RequirementInfo={} %GIDa_11e886ba_5fe6_4535_bddc_cd68d6707c0e  Port=11  InitialOutput=0
  u8AdaptiveCurrentIndex : Outport  RequirementInfo={} %GIDa_63caae96_ca96_48de_8688_67b8bf167e40  Port=12  InitialOutput=0
  bIsMvtBeltControlled : Outport  RequirementInfo={} %GIDa_d0ae1f82_bdf1_4e59_a7de_1b923e4044a1  Port=13  InitialOutput=0
  bBeltPayoutAbortion2 : Outport  RequirementInfo={} %GIDa_beb02f68_2905_400f_b8cc_508588365440  Port=14  InitialOutput=0
  bBeltPayoutAbortion1 : Outport  RequirementInfo={} %GIDa_66eafeda_0478_4345_9518_2634965f68e3  Port=15  InitialOutput=0
  wires:
  In14/1 -> bIsMvtBeltControlled/1
  In13/1 -> u8AdaptiveCurrentIndex/1
  In12/1 -> eCurrentRegulationType/1
  In10/1 -> bBeltBlockedControlled/1
  In9/1 -> bWeightedStep/1
  In8/1 -> bRampStep/1
  In7/1 -> bOrderControlled/1
  In6/1 -> bReleasedControlled/1
  In5/1 -> bMotorBlockedControlled/1
  In4/1 -> bTrigOffControlled/1
  In3/1 -> u16StepDuration/1
  In2/1 -> s8OrderValue/1
  In1/1 -> u8OrderType/1
  In11/1 -> bBeltPayoutAbortion2/1
  In15/1 -> bBeltPayoutAbortion1/1

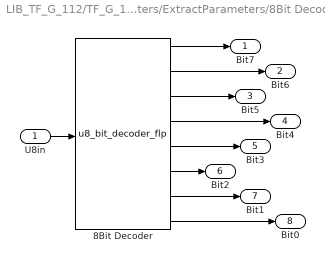
== system LIB_TF_G_112/TF_G_112/Manage Step Parameters/ExtractParameters/8Bit Decoder ==
  U8in : Inport  RequirementInfo={} %GIDa_316296e6_d25f_415d_86a4_ab2f303f2967
  8Bit Decoder : S-Function  RequirementInfo={} %GIDa_81db60bf_2ae0_4350_8dba_f94edd03fe1c  FunctionName=u8_bit_decoder_flp  Parameters=dt  SFunctionDeploymentMode=off  EnableBusSupport=off  mask(TL_CustomCode){data={'#state',0,'#param',0,'#work',0,'#output',8,'#logdata',8,'codefile','u8_bit_decoder.c','output#1',{'name','bIsRampStepRaw','varname','bit7','type','Bool'},'output#2',{'name','$S_$B_bit6','varname','bit6','type','Bool'},'output#3',{'name','bIsReleaseCtrlRaw','varname','bit5','type','Bool'},'output#4',{'name','$S_$B_bit4','varname','bit4','type','Bool'},'output#5',{'name','$S_$B_bit3','varname','bit3','type','Bool'},'output#6',{'name','$S_$B_bit2','varname','bit2','type','Bool'},'output#7',{'name','$S_$B_bit1','varname','bit1','type','Bool'},'output#8',{'name','$S_$B_bit0','varname','bit0','type','Bool'},'input',{'name','$S_$B_in','varname','u8in','type','UInt8'},'date',735951.66829136573}, dt=-1}
      mask help:
      | TargetLink Custom Code block:
      | Allows to insert custom code into a TargetLink application.
      settings: DeleteFcn=if exist('delete_tlblock','file')==2,delete_tlblock(gcbh);end  NameChangeFcn=if exist('rename_tlblock','file')==2,rename_tlblock(gcbh);end  OpenFcn=if exist('tl_open_blockdlg','file')==2,tl_open_blockdlg(gcbh);else,open_system(gcbh,'mask');end
      mask Help: eval('if exist(''tl_online_help'',''file'') == 2, tl_online_help(''Topic'',get_param(gcbh,''MaskType'')),end')
      mask Display:
      | plot([-0.05, 1.05, NaN, -0.05, 1.05],[.01, .01, NaN, .99, .99])
      | ; disp('u8_bit_decoder.c');port_label('input',1,'u8in');port_label('output',1,'bit7');port_label('output',2,'bit6');port_label('output',3,'bit5');port_label('output',4,'bit4');port_label('output',5,'bit3');port_label('output',6,'bit2');port_label('output',7,'bit1');port_label('output',8,'bit0');
  Bit7 : Outport  RequirementInfo={} %GIDa_3e1253f0_2b66_4f5f_9a2b_0a84a073a355
  Bit6 : Outport  RequirementInfo={} %GIDa_a627d821_e196_4b9f_ab67_4eedadb88607  Port=2
  Bit5 : Outport  RequirementInfo={} %GIDa_63315573_79b3_40d9_a8a2_9d817ae078b8  Port=3
  Bit4 : Outport  RequirementInfo={} %GIDa_f646e766_972f_4fff_a2f4_989fa47cfa97  Port=4
  Bit3 : Outport  RequirementInfo={} %GIDa_8223dec1_0264_454d_b26b_ef6deaf87ddf  Port=5
  Bit2 : Outport  RequirementInfo={} %GIDa_adc812c1_ffaa_4134_971e_8e5418b5c1d2  Port=6
  Bit1 : Outport  RequirementInfo={} %GIDa_18117852_57bb_4938_bdc2_0ce63c214a6d  Port=7
  Bit0 : Outport  RequirementInfo={} %GIDa_201e9e1e_c2ed_40b8_a640_dde971076c79  Port=8
  wires:
  U8in/1 -> 8Bit Decoder/1
  8Bit Decoder/6 -> Bit2/1
  8Bit Decoder/1 -> Bit7/1
  8Bit Decoder/2 -> Bit6/1
  8Bit Decoder/3 -> Bit5/1
  8Bit Decoder/4 -> Bit4/1
  8Bit Decoder/5 -> Bit3/1
  8Bit Decoder/7 -> Bit1/1
  8Bit Decoder/8 -> Bit0/1

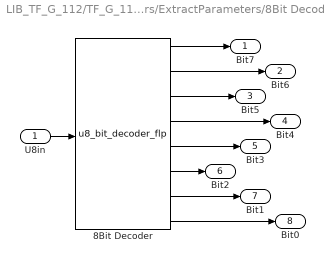
== system LIB_TF_G_112/TF_G_112/Manage Step Parameters/ExtractParameters/8Bit Decoder1 ==
  U8in : Inport  RequirementInfo={} %GIDa_2453706d_6a1d_4b38_b9bc_9d9f68181e7c
  8Bit Decoder : S-Function  RequirementInfo={} %GIDa_3ecb15fb_eb47_429a_8f6b_68399114027c  FunctionName=u8_bit_decoder_flp  Parameters=dt  SFunctionDeploymentMode=off  EnableBusSupport=off  mask(TL_CustomCode){data={'#state',0,'#param',0,'#work',0,'#output',8,'#logdata',8,'codefile','u8_bit_decoder.c','output#1',{'variable','Internal_Interfaces/bUnusedDecoder8Bits','varname','bit7'},'output#2',{'variable','Internal_Interfaces/bUnusedDecoder8Bits','varname','bit6'},'output#3',{'name','bIsBeltBlockedRaw','varname','bit5','type','Bool'},'output#4',{'name','$S_$B_bit4','varname','bit4','type','Bool'},'output#5',{'name','bIsBeltMvtRaw','varname','bit3','type','Bool'},'output#6',{'name','bIsBeltPayoutAbortion2','varname','bit2','type','Bool'},'output#7',{'name','bIsBeltPayoutAbortion1','varname','bit1','type','Bool'},'output#8',{'name','bIsHighPowerSet','varname','bit0','type','Bool'},'input',{'name','$S_$B_in','varname','u8in','type','UInt8'},'date',735951.66828944441}, dt=-1}
      mask help:
      | TargetLink Custom Code block:
      | Allows to insert custom code into a TargetLink application.
      settings: DeleteFcn=if exist('delete_tlblock','file')==2,delete_tlblock(gcbh);end  NameChangeFcn=if exist('rename_tlblock','file')==2,rename_tlblock(gcbh);end  OpenFcn=if exist('tl_open_blockdlg','file')==2,tl_open_blockdlg(gcbh);else,open_system(gcbh,'mask');end
      mask Help: eval('if exist(''tl_online_help'',''file'') == 2, tl_online_help(''Topic'',get_param(gcbh,''MaskType'')),end')
      mask Display:
      | plot([-0.05, 1.05, NaN, -0.05, 1.05],[.01, .01, NaN, .99, .99])
      | ; disp('u8_bit_decoder.c');port_label('input',1,'u8in');port_label('output',1,'bit7');port_label('output',2,'bit6');port_label('output',3,'bit5');port_label('output',4,'bit4');port_label('output',5,'bit3');port_label('output',6,'bit2');port_label('output',7,'bit1');port_label('output',8,'bit0');
  Bit7 : Outport  RequirementInfo={} %GIDa_37ae538e_3b26_4c9d_a1b0_9161462b1858
  Bit6 : Outport  RequirementInfo={} %GIDa_073366e0_0148_498b_90f8_a0f7c3e501ce  Port=2
  Bit5 : Outport  RequirementInfo={} %GIDa_27038c08_5069_4df1_b6c4_3a6e681f6bef  Port=3
  Bit4 : Outport  RequirementInfo={} %GIDa_35cce3eb_b6ca_4f36_956e_9ba57a31904a  Port=4
  Bit3 : Outport  RequirementInfo={} %GIDa_6a1f7b1a_7853_4efa_9eab_a071e8e9086b  Port=5
  Bit2 : Outport  RequirementInfo={} %GIDa_0127094a_cacc_4da3_8246_4af2c1ed6524  Port=6
  Bit1 : Outport  RequirementInfo={} %GIDa_e068d61d_7382_40af_ae73_e21953aa876a  Port=7
  Bit0 : Outport  RequirementInfo={} %GIDa_f4ec7002_3337_4088_8267_904cc4e0ca7c  Port=8
  wires:
  8Bit Decoder/8 -> Bit0/1
  8Bit Decoder/7 -> Bit1/1
  8Bit Decoder/5 -> Bit3/1
  8Bit Decoder/4 -> Bit4/1
  8Bit Decoder/3 -> Bit5/1
  8Bit Decoder/2 -> Bit6/1
  8Bit Decoder/1 -> Bit7/1
  8Bit Decoder/6 -> Bit2/1
  U8in/1 -> 8Bit Decoder/1

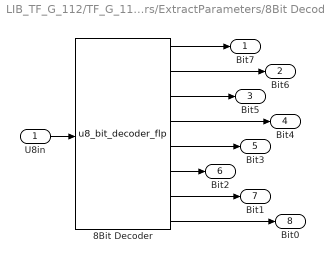
== system LIB_TF_G_112/TF_G_112/Manage Step Parameters/ExtractParameters/8Bit Decoder2 ==
  U8in : Inport  RequirementInfo={} %GIDa_045b19ce_b7c1_41cb_92f1_8e22c3213688
  8Bit Decoder : S-Function  RequirementInfo={} %GIDa_b7b0766f_5ee3_49a7_9996_d49378d69685  FunctionName=u8_bit_decoder_flp  Parameters=dt  SFunctionDeploymentMode=off  EnableBusSupport=off  mask(TL_CustomCode){data={'#state',0,'#param',0,'#work',0,'#output',8,'#logdata',8,'codefile','u8_bit_decoder.c','output#1',{'variable','Internal_Interfaces/bUnusedDecoder8Bits','varname','bit7'},'output#2',{'variable','Internal_Interfaces/bUnusedDecoder8Bits','varname','bit6'},'output#3',{'variable','Internal_Interfaces/bUnusedDecoder8Bits','varname','bit5'},'output#4',{'variable','Internal_Interfaces/bUnusedDecoder8Bits','varname','bit4'},'output#5',{'variable','Internal_Interfaces/bUnusedDecoder8Bits','varname','bit3'},'output#6',{'variable','Internal_Interfaces/bUnusedDecoder8Bits','varname','bit2'},'output#7',{'name','bIsPidMotorSet','varname','bit1','type','Bool'},'output#8',{'name','bIsPidBatterySet','varname','bit0','type','Bool'},'input',{'name','$S_$B_in','varname','u8in','type','UInt8'},'date',735951.66828739585}, dt=-1}
      mask help:
      | TargetLink Custom Code block:
      | Allows to insert custom code into a TargetLink application.
      settings: DeleteFcn=if exist('delete_tlblock','file')==2,delete_tlblock(gcbh);end  NameChangeFcn=if exist('rename_tlblock','file')==2,rename_tlblock(gcbh);end  OpenFcn=if exist('tl_open_blockdlg','file')==2,tl_open_blockdlg(gcbh);else,open_system(gcbh,'mask');end
      mask Help: eval('if exist(''tl_online_help'',''file'') == 2, tl_online_help(''Topic'',get_param(gcbh,''MaskType'')),end')
      mask Display:
      | plot([-0.05, 1.05, NaN, -0.05, 1.05],[.01, .01, NaN, .99, .99])
      | ; disp('u8_bit_decoder.c');port_label('input',1,'u8in');port_label('output',1,'bit7');port_label('output',2,'bit6');port_label('output',3,'bit5');port_label('output',4,'bit4');port_label('output',5,'bit3');port_label('output',6,'bit2');port_label('output',7,'bit1');port_label('output',8,'bit0');
  Bit7 : Outport  RequirementInfo={} %GIDa_69e05ae1_626f_4283_965b_4c833d7b5f3e
  Bit6 : Outport  RequirementInfo={} %GIDa_bcb75647_8ceb_46a2_bba2_e67bcad83520  Port=2
  Bit5 : Outport  RequirementInfo={} %GIDa_71d0168b_9fc1_4d93_b3be_8e57ddf94a21  Port=3
  Bit4 : Outport  RequirementInfo={} %GIDa_3921d2bc_78ab_4767_b043_ff960ee36e30  Port=4
  Bit3 : Outport  RequirementInfo={} %GIDa_f5b9b550_7a96_427c_8ba3_eed7ce10c758  Port=5
  Bit2 : Outport  RequirementInfo={} %GIDa_4a7fd827_c97b_4016_8ff5_91849af033ba  Port=6
  Bit1 : Outport  RequirementInfo={} %GIDa_9b34eff2_06c8_4b9c_9ba5_cc0515da6db3  Port=7
  Bit0 : Outport  RequirementInfo={} %GIDa_3d9e95a2_fc52_4db0_bcb3_e6c8f2579aa8  Port=8
  wires:
  U8in/1 -> 8Bit Decoder/1
  8Bit Decoder/6 -> Bit2/1
  8Bit Decoder/1 -> Bit7/1
  8Bit Decoder/2 -> Bit6/1
  8Bit Decoder/3 -> Bit5/1
  8Bit Decoder/4 -> Bit4/1
  8Bit Decoder/5 -> Bit3/1
  8Bit Decoder/7 -> Bit1/1
  8Bit Decoder/8 -> Bit0/1
